simulink model "delay_track_fshift_sim"  (R2019a)
settings: Solver=VariableStepAuto  StartTime=0.0  StopTime=500000 / (fs_ghz * 1e9)  RelTol=1e-3
undefined symbols (not defined in the file or in its folder): fdesignblkfcn, fs_ghz, gcbh
libraries: dspmtrx3 x5, dspxfrm3 x2, simulink x1
(part 5 of 7)

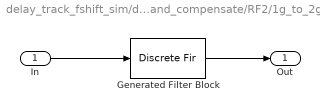
== system delay_track_fshift_sim/delay_and_compensate/RF2/1g_to_2g_filt ==
  In : Inport
  Generated Filter Block : DiscreteFir  Tag=BlockMethodSubSystem  Coefficients=[1.01704780809032204e-05 8.00513267945117663e-06 5.63585570426750819e-06 3.08357437286688761e-06 3.7215072795178805e-07 -2.47188488010559091e-06 -5.41963823333738916e-06 -8.44018986497744443e-06 -1.15009636491456078e-05 -1.45681207425512571e-05 -1.76069739067568088e-05 -2.05824169501533862e-05 -2.34593638064728185e-05 -2.62031916145401389e-05 -2.87801820842337675e-05 -3.11579554275093182e-05 -3.33058912012263827e-05 -3.51955305497911027e-05 -3.68009545486803872e-05 -3.80991336323416313e-05 -3.90702434383280797e-05 -3.9697942809654596e-05 -3.99696101641509923e-05 -3.98765349573121543e-05 -3.9414061527323254e-05 -3.85816832105021653e-05 -3.73830852448271656e-05 -3.58261356305002515e-05 -3.39228237813690925e-05 -3.16891474709768238e-05 -2.91449492434603356e-05 -2.63137041138389541e-05 -2.32222610159979108e-05 -1.99005410615876088e-05 -1.63811962412235288e-05 -1.26992327233049705e-05 -8.8916033785218103e-06 -4.99677457331138471e-06 -1.05427262762551766e-06 2.8957843835481494e-06 6.81316359336166254e-06 1.06579970423668198e-05 1.43912580253996491e-05 1.79752280161215783e-05 2.13739481962684946e-05 2.45536497913099621e-05 2.74831576646563119e-05 3.01342619459547984e-05 3.24820528615073857e-05 3.45052143917845336e-05 3.61862728967662627e-05 3.75117974180645976e-05 3.84725489803801237e-05 3.90635768661212252e-05 3.92842605176785885e-05 3.91382964232687674e-05 3.86336300554014343e-05 3.77823336466940522e-05 3.66004312966416659e-05 3.51076735957998195e-05 3.33272646214891172e-05 3.12855447927819211e-05 2.90116336636708857e-05 2.65370372739731335e-05 2.38952251603562046e-05 2.11211825481871986e-05 1.82509435928104951e-05 1.53211118114295384e-05 1.23683740398709561e-05 9.42901435918388826e-06 6.53843446321893443e-06 3.73068687922617227e-06 1.03802730927193963e-06 -1.50950786776733833e-06 -3.88449320321778217e-06 -6.06246955139397891e-06 -8.02225832534259662e-06 -9.74623028080327068e-06 -1.12205250628871434e-05 -1.24352183930316817e-05 -1.33844344625079767e-05 -1.40664018243934819e-05 -1.44834518290852903e-05 -1.46419594193680697e-05 -1.4552226879642693e-05 -1.42283119099223237e-05 -1.36878021582127459e-05 -1.29515390847462033e-05 -1.20432947381423258e-05 -1.0989405687273203e-05 -9.81836896423527479e-06 -8.56040542477295611e-06 -7.24699641493717604e-06 -5.91040003964795905e-06 -4.58315365413278197e-06 -3.29756943787173283e-06 -2.08523005871698283e-06 -9.76491489596542044e-07 6.95422859358966016e-19 8.17769790987127885e-07 1.45294914298243821e-06 1.88467536857455149e-06 2.09545202846574502e-06 2.0714637166031498e-06 1.80284057665941826e-06 1.28386833457933286e-06 5.13140338449350565e-07 -5.06351142251884032e-07 -1.76718630053984656e-06 -3.25755296183558561e-06 -4.96134577986520644e-06 -6.85832882365886468e-06 -8.92436004562925597e-06 -1.11316752570225396e-05 -1.34492283965289128e-05 -1.58430840720695005e-05 -1.82768575958664113e-05 -2.07121970296069048e-05 -2.31093011198088888e-05 -2.54274664427061037e-05 -2.76256566013520524e-05 -2.96630859325334825e-05 -3.14998098936618306e-05 -3.30973141148823509e-05 -3.44190940228807595e-05 -3.543121697243807e-05 -3.61028589604328658e-05 -3.6406808244058192e-05 -3.63199285383882368e-05 -3.58235749244140784e-05 -3.49039561523819891e-05 -3.35524376702317555e-05 -3.17657804355690599e-05 -2.95463113729608637e-05 -2.690202220653732e-05 -2.38465943198959583e-05 -2.03993482593982608e-05 -1.65851174906108865e-05 -1.24340470278901964e-05 -7.98131857053603501e-06 -3.26680478202306088e-06 1.66534367209683915e-06 6.76717377022089742e-06 1.19874630158975112e-05 1.72723032769409683e-05 2.256572855146389e-05 2.78103789616575999e-05 3.29481927035480009e-05 3.79211172126135961e-05 4.26718304484472103e-05 4.7144462962604513e-05 5.128531129692916e-05 5.50435332677490927e-05 5.83718158257775737e-05 6.12270064417469586e-05 6.35706993517340244e-05 6.53697684998394798e-05 6.65968396340070536e-05 6.72306947361180724e-05 6.72566027915482654e-05 6.66665718160618689e-05 6.54595180479316581e-05 6.36413492680329754e-05 ...(+56527 chars)]  InputProcessing=Columns as channels (frame based)
  Out : Outport
  wires:
  In/1 -> Generated Filter Block/1
  Generated Filter Block/1 -> Out/1
